simulink model "BMS_V4"  (R2017b)
settings: Solver=FixedStepDiscrete  StartTime=0.0  StopTime=inf  FixedStep=BASETIME  RelTol=1e-3  EnableMultiTasking=on
values from neighbouring files (symbols this model uses):
  AKT_BALANCE = uint16(8)    [BMS_V4_config.m]
  BALANCE = uint16(4)    [BMS_V4_config.m]
  BALANCE_RESISTOR = int32(5)    [BMS_V4_config.m]
  BALANCE_VEC = uint16(8)    [BMS_V4_config.m]
  CELL_SOC = uint16(7)    [BMS_V4_config.m]
  CELL_STATE = uint16(3)    [BMS_V4_config.m]
  CELL_TEMPERATURE = uint16(6)    [BMS_V4_config.m]
  CELL_VOLTAGE = uint16(5)    [BMS_V4_config.m]
  CELLACTBITFIELD = hex2dec('300')    [BMS_V4_config.m]
  CELLDEACTBITFIELD = hex2dec('100')    [BMS_V4_config.m]
  CELLT_BURST = uint16(6)    [BMS_V4_config.m]
  CELLV_BURST = uint16(5)    [BMS_V4_config.m]
  CLK_CYC_timer_1 = 586    [BMS_V4_config.m]
  CLK_CYC_timer_2 = 5860    [BMS_V4_config.m]
  CLK_CYC_timer_3 = 280    [BMS_V4_config.m]
  CLK_CYC_timer_4 = 586*100    (= 58600)    [BMS_V4_config.m]
  CLK_CYC_timer_5 = 5800*2    (= 11600)    [BMS_V4_config.m]
  CLK_CYC_timer_6 = 320    [BMS_V4_config.m]
  CN_CELLS = int32(40*3600)    [BMS_V4_config.m]
  CONTACTOR = uint16(1)    [BMS_V4_config.m]
  CONTACTOR_LOCKED = uint16(0)    [BMS_V4_config.m]
  CONTACTOR_UNLOCKED = uint16(1)    [BMS_V4_config.m]
  DEBUG_SEND_STATES = uint16(hex2dec('01'))    [BMS_V4_config.m]
  DELTA_SOC_BALANCE = int32(5*1e6)    [BMS_V4_config.m]
  DELTA_SOC_BALANCE_OFF = int32(1*1e5)    [BMS_V4_config.m]
  DETERMINE_MODEL_PARAMETER_ACT = uint16(100)    [BMS_V4_config.m]
  DETERMINE_MODEL_PARAMETER_SCC = uint16(101)    [BMS_V4_config.m]
  ERROR = uint16(1)    [BMS_V4_config.m]
  EXTERN_SIGNALS = uint16(1)    [BMS_V4_config.m]
  FREQUENCY_STEPS = uint16([25 50 75 100 150 250 500 750                                      1000 1500 2500 5000 7500                                      10010 10015 10025 10050 10075                                      10100 10150 10250 10500 10750                                      11000 11500])    [BMS_V4_config.m]
  GET_IMAG_PART_MFC = uint16(9)    [BMS_V4_config.m]
  GET_IMAG_PART_MSF = uint16(4)    [BMS_V4_config.m]
  GET_REAL_PART_MFC = uint16(8)    [BMS_V4_config.m]
  GET_REAL_PART_MSF = uint16(3)    [BMS_V4_config.m]
  IMU = uint16(7)    [BMS_V4_config.m]
  IMU_AMP_OFF = uint16(5)    [BMS_V4_config.m]
  IMU_DATA_READ_LOCUS_ACT = uint16(6)    [BMS_V4_config.m]
  IMU_DATA_READ_LOCUS_SCC = uint16(7)    [BMS_V4_config.m]
  IMU_DEBUG = uint16(9)    [BMS_V4_config.m]
  IMU_GET_DATA_MFC = uint16(8)    [BMS_V4_config.m]
  IMU_GET_DATA_MSF = uint16(3)    [BMS_V4_config.m]
  IMU_OFFSET_POLLING = uint16(11)    [BMS_V4_config.m]
  IMU_POLLING = uint16(2)    [BMS_V4_config.m]
  IMU_POWER = uint16(10)    [BMS_V4_config.m]
  IMU_SEND_IMAG = uint16(11)    [BMS_V4_config.m]
  IMU_SEND_REAL = uint16(10)    [BMS_V4_config.m]
  INDEX_IMAGPART = uint16(2)    [BMS_V4_config.m]
  INDEX_REALPART = uint16(1)    [BMS_V4_config.m]
  INFO = uint16(2)    [BMS_V4_config.m]
  INIT_OFFSET_AMPLITUDE = uint16(2)    [BMS_V4_config.m]
  LINE_CURRENT = uint16(3)    [BMS_V4_config.m]
  LINE_CURRENT_CANA = uint16(4)    [BMS_V4_config.m]
  LINE_CURRENT_SWITCH_THRESHOLD = int32(2*1e6)    [BMS_V4_config.m]
  NUM_OF_CELLS = uint16(16)    [BMS_V4_config.m]
  NUM_OF_FREQUENCIES_PSO = uint16(14)    [BMS_V4_config.m]
  NUM_OF_LINES = uint16(1)    [BMS_V4_config.m]
  NUM_OF_PARAMETER = single(5)    [BMS_V4_config.m]
  NUM_OF_SOC_POINTS = uint16(110)    [BMS_V4_config.m]
  P_L_BOUND = single([0.05;0.01;0.1;0.01;0.1])    [BMS_V4_config.m]
  P_U_BOUND = single([0.50;0.20;0.9;0.06;60])    [BMS_V4_config.m]
  PARA_ACT_SEND = uint16(101)    [BMS_V4_config.m]
  PARA_DATA_STORE_ACT = uint16(8)    [BMS_V4_config.m]
  PARA_DATA_STORE_SCC = uint16(9)    [BMS_V4_config.m]
  PARA_SCC_SEND = uint16(102)    [BMS_V4_config.m]
  PARTICLE_INIT = single(create_startparticle(P_L_BOUND,P_U_BOUND,NUM_OF_PARTICLE))    [BMS_V4_config.m]
  POLACT = hex2dec('00000BFF')    [BMS_V4_config.m]
  POLDEACT = hex2dec('000008FF')    [BMS_V4_config.m]
  PSO_PARA_DEBUG = uint16(13)    [BMS_V4_config.m]
  REQUEST_SOC_REF = uint16(1000)    [BMS_V4_config.m]
  SCALE_FACTOR_CH1 = single(0.66666666)    [BMS_V4_config.m]
  SCALE_FACTOR_CH2 = single(0.66666666)    [BMS_V4_config.m]
  SEND_CELL_SOC_ABS = uint16(199)    [BMS_V4_config.m]
  SHUT_DOWN_BALANCE_OFF = uint16(3)    [BMS_V4_config.m]
  SHUT_DOWN_BALANCE_ON = uint16(2)    [BMS_V4_config.m]
  START_IMU_MSL = uint16(3)    [BMS_V4_config.m]
  START_IMU_SCC = uint16(1)    [BMS_V4_config.m]
  SWITCH_IMU_OFF = uint16(2)    [BMS_V4_config.m]
  SWITCH_IMU_ON = uint16(1)    [BMS_V4_config.m]
  SWITCH_IMU_ON_OFF = uint16(4)    [BMS_V4_config.m]
  SYSTEM_DEBUG = uint16(12)    [BMS_V4_config.m]
  TIMEOUT_CANA = uint32(5000)    [BMS_V4_config.m]
  TIMEOUT_GATEWAY = uint32(500)    [BMS_V4_config.m]
  TS_SOC = single(0.010)    [BMS_V4_config.m]
  WARNING = uint16(2)    [BMS_V4_config.m]
libraries: c280xlib x44, c2833xlib x5, simulink x2, c2000lib x1, idelinklib_common x1
(part 1 of 8)
settings Model: Creator=Rathmann  LastModifiedBy=Franke
settings DataIOCC: LimitDataPoints=on  SaveFormat=Array
settings OptimizationCC: DefaultUnderspecifiedDataType=single  LifeSpan=1  MaxStackSize=64
settings DebuggingCC: SolverPrmCheckMsg=warning  MultiTaskDSMMsg=warning  AllowSymbolicDim=off  SFUnexpectedBacktrackingDiag=warning  SFNoUnconditionalDefaultTransitionDiag=warning  SFExecutionAtInitializationDiag=none
settings HardwareCC: ProdBitPerChar=16  ProdBitPerInt=16  ProdBitPerPointer=16  ProdBitPerSizeT=32  ProdBitPerPtrDiffT=32  ProdLargestAtomicInteger=Integer  ProdLargestAtomicFloat=None  ProdWordSize=16  ProdHWDeviceType=Texas Instruments->C2000
settings ModelReferenceCC: PropagateSignalLabelsOutOfModel=off
settings SFSimCC: MATLABDynamicMemAlloc=off
settings RTWCC: SystemTargetFile=ert.tlc  HardwareBoard=TI Delfino F2833x (boot from flash)  TLCOptions=-aInlineSetEventsForThisBaseRateFcn=TLC_FALSE -aSuppressMultiTaskScheduler=TLC_FALSE -aRateBasedStepFcn=1  TemplateMakefile=ert_default_tmf  RTWVerbose=off  Toolchain=Texas Instruments Code Composer Studio (C2000)  BuildConfiguration=Faster Runs
settings CodeAppCC: IgnoreCustomStorageClasses=off  StateflowObjectComments=on
settings ERTTargetCC: CodeReplacementLibrary=TI C28x with C99 extensions  MultiwordLength=2048  CombineOutputUpdateFcns=off  ConvertIfToSwitch=off  SuppressUnreachableDefaultCases=off  MemSecPackage=mpt
settings ConfigComp: CovMetricSettings=dw  CovHtmlReporting=on  CovSaveCumulativeToWorkspaceVar=on  CovSaveSingleToWorkspaceVar=on  CovExternalEMLEnable=off  CovSFcnEnable=off

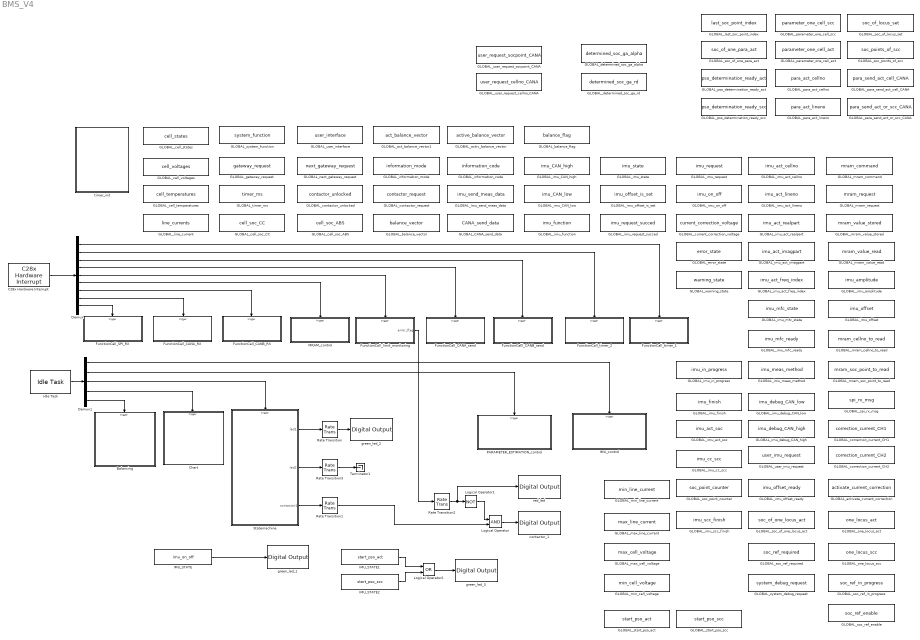
== system BMS_V4 ==
  Balancing : Stateflow chart  TreatAsAtomicUnit=on
  C28x Hardware Interrupt : c2000lib/Scheduling/C28x Hardware Interrupt  irqnumbers=[3 3 3 3 3 3 9 9 6]  pienumbers=[1 2 3 4 5 6 7 6 1]  irqpriorities=[36 37 38 39 30 41 35 34 33]  irqpreempts=[0 0 0 0 0 0 0 0 0]  showinput=off  dspchiptype=C280X
      settings: SourceProductName=Embedded Coder Support Package for Texas Instruments C2000 Processors  SourceProductBaseCode=TIC2000
  Chart : Stateflow chart  TreatAsAtomicUnit=on
  Demux : Demux  Outputs=9
  Demux1 : Demux  Outputs=5
  FunctionCall_CANA_RX : Subsystem  TreatAsAtomicUnit=on
      settings: RTWSystemCode=Nonreusable function  RTWFcnNameOpts=Use subsystem name  RTWFileNameOpts=Use subsystem name
  FunctionCall_CANA_send : Subsystem  TreatAsAtomicUnit=on
      settings: RTWSystemCode=Nonreusable function  RTWFcnNameOpts=Use subsystem name  RTWFileNameOpts=Use subsystem name
  FunctionCall_CANB_RX : Subsystem  TreatAsAtomicUnit=on
      settings: RTWSystemCode=Nonreusable function  RTWFcnNameOpts=Use subsystem name  RTWFileNameOpts=Use subsystem name  FunctionInterfaceSpec=Allow arguments
  FunctionCall_SPI_RX : Subsystem  TreatAsAtomicUnit=on
      settings: RTWSystemCode=Nonreusable function  RTWFcnNameOpts=Use subsystem name  RTWFileNameOpts=Use subsystem name
  FunctionCall_limit_monitoring : Stateflow chart  TreatAsAtomicUnit=on
      settings: RTWSystemCode=Nonreusable function  RTWFcnNameOpts=Use subsystem name  RTWFileNameOpts=Use subsystem name
  FunctionCall_timer_1 : Subsystem  TreatAsAtomicUnit=on
      settings: RTWSystemCode=Nonreusable function  RTWFcnNameOpts=Use subsystem name  RTWFileNameOpts=Use subsystem name
  FunctionCall_timer_2 : Subsystem  TreatAsAtomicUnit=on
      settings: RTWSystemCode=Nonreusable function  RTWFcnNameOpts=Use subsystem name  RTWFileNameOpts=Use subsystem name  FunctionInterfaceSpec=Allow arguments
  FunctionCalll_CANB_send : Subsystem  TreatAsAtomicUnit=on
      settings: RTWSystemCode=Nonreusable function  RTWFcnNameOpts=Use subsystem name  RTWFileNameOpts=Use subsystem name
  GLOBAL_CANA_send_data : DataStoreMemory  DataStoreName=CANA_send_data  ReadBeforeWriteMsg=warning  WriteAfterWriteMsg=warning  WriteAfterReadMsg=warning  InitialValue=CANA_SEND_DATA_INIT  ShowAdditionalParam=off  OutDataTypeStr=boolean
  GLOBAL_act_balance_vector1 : DataStoreMemory  DataStoreName=act_balance_vector  ReadBeforeWriteMsg=warning  WriteAfterWriteMsg=warning  WriteAfterReadMsg=warning  InitialValue=BALANCE_VECTOR_INIT  ShowAdditionalParam=off  OutDataTypeStr=boolean
  GLOBAL_activ_balance_vector : DataStoreMemory  DataStoreName=active_balance_vector  ReadBeforeWriteMsg=warning  WriteAfterWriteMsg=warning  WriteAfterReadMsg=warning  InitialValue=ACTIVE_BALANCE_VECTOR_INIT  ShowAdditionalParam=off  OutDataTypeStr=uint32
  GLOBAL_activate_current_correction : DataStoreMemory  DataStoreName=activate_current_correction  ReadBeforeWriteMsg=warning  WriteAfterWriteMsg=warning  WriteAfterReadMsg=warning  ShowAdditionalParam=off  OutDataTypeStr=boolean
  GLOBAL_balance_flag : DataStoreMemory  DataStoreName=balance_flag  ReadBeforeWriteMsg=warning  WriteAfterWriteMsg=warning  WriteAfterReadMsg=warning  InitialValue=BALANCE_FLAG_INIT  ShowAdditionalParam=off  OutDataTypeStr=boolean
  GLOBAL_balance_vector : DataStoreMemory  DataStoreName=balance_vector  ReadBeforeWriteMsg=warning  WriteAfterWriteMsg=warning  WriteAfterReadMsg=warning  InitialValue=BALANCE_VECTOR_INIT  ShowAdditionalParam=off  OutDataTypeStr=boolean
  GLOBAL_cell_soc_ABS : DataStoreMemory  DataStoreName=cell_soc_ABS  ReadBeforeWriteMsg=warning  WriteAfterWriteMsg=warning  WriteAfterReadMsg=warning  InitialValue=CELL_SOC_ABS_INIT  ShowAdditionalParam=off  OutDataTypeStr=int32
  GLOBAL_cell_soc_CC : DataStoreMemory  DataStoreName=cell_soc_CC  ReadBeforeWriteMsg=warning  WriteAfterWriteMsg=warning  WriteAfterReadMsg=warning  InitialValue=CELL_SOC_CC_INIT  ShowAdditionalParam=off  OutDataTypeStr=int32
  GLOBAL_cell_states : DataStoreMemory  DataStoreName=cell_states  ReadBeforeWriteMsg=warning  WriteAfterWriteMsg=warning  WriteAfterReadMsg=warning  InitialValue=CELL_STATES_INIT  ShowAdditionalParam=off  OutDataTypeStr=uint32  DataLoggingName=va
      settings: DataLoggingNameMode=Custom
  GLOBAL_cell_temperatures : DataStoreMemory  DataStoreName=cell_temperatures  ReadBeforeWriteMsg=warning  WriteAfterWriteMsg=warning  WriteAfterReadMsg=warning  InitialValue=CELL_TEMPERATURES_INIT  VectorParams1D=off  ShowAdditionalParam=off  OutDataTypeStr=int16
  GLOBAL_cell_voltages : DataStoreMemory  DataStoreName=cell_voltages  ReadBeforeWriteMsg=warning  WriteAfterWriteMsg=warning  WriteAfterReadMsg=warning  InitialValue=CELL_VOLTAGES_INIT  ShowAdditionalParam=off  OutDataTypeStr=uint16  DataLoggingName=va
      settings: DataLoggingNameMode=Custom
  GLOBAL_contactor_request : DataStoreMemory  DataStoreName=contactor_request  ReadBeforeWriteMsg=warning  WriteAfterWriteMsg=warning  WriteAfterReadMsg=warning  ShowAdditionalParam=off  OutDataTypeStr=boolean
  GLOBAL_contactor_unlocked : DataStoreMemory  DataStoreName=contactor_unlocked  ReadBeforeWriteMsg=warning  WriteAfterWriteMsg=warning  WriteAfterReadMsg=warning  ShowAdditionalParam=off  OutDataTypeStr=boolean
  GLOBAL_correction_current_CH1 : DataStoreMemory  DataStoreName=correction_current_CH1  ReadBeforeWriteMsg=warning  WriteAfterWriteMsg=warning  WriteAfterReadMsg=warning  InitialValue=CURRENT_CORRECTION_INIT  ShowAdditionalParam=off  OutDataTypeStr=single
  GLOBAL_correction_current_CH2 : DataStoreMemory  DataStoreName=correction_current_CH2  ReadBeforeWriteMsg=warning  WriteAfterWriteMsg=warning  WriteAfterReadMsg=warning  InitialValue=CURRENT_CORRECTION_INIT  ShowAdditionalParam=off  OutDataTypeStr=single
  GLOBAL_current_correction_voltage : DataStoreMemory  DataStoreName=current_correction_voltage  ReadBeforeWriteMsg=warning  WriteAfterWriteMsg=warning  WriteAfterReadMsg=warning  ShowAdditionalParam=off  OutDataTypeStr=uint16
  GLOBAL_determined_soc_ga_alpha : DataStoreMemory  DataStoreName=determined_soc_ga_alpha  ReadBeforeWriteMsg=warning  WriteAfterWriteMsg=warning  WriteAfterReadMsg=warning  InitialValue=DETERMINED_SOC_GA_INIT  ShowAdditionalParam=off  OutDataTypeStr=int32
  GLOBAL_determined_soc_ga_rd : DataStoreMemory  DataStoreName=determined_soc_ga_rd  ReadBeforeWriteMsg=warning  WriteAfterWriteMsg=warning  WriteAfterReadMsg=warning  InitialValue=DETERMINED_SOC_GA_INIT  ShowAdditionalParam=off  OutDataTypeStr=int32
  GLOBAL_error_state : DataStoreMemory  DataStoreName=error_state  ReadBeforeWriteMsg=warning  WriteAfterWriteMsg=warning  WriteAfterReadMsg=warning  InitialValue=[0 0]  ShowAdditionalParam=off  OutDataTypeStr=uint16
  GLOBAL_gateway_request : DataStoreMemory  DataStoreName=gateway_request  ReadBeforeWriteMsg=warning  WriteAfterWriteMsg=warning  WriteAfterReadMsg=warning  InitialValue=GATEWAY_REQUEST_INIT  ShowAdditionalParam=off  OutDataTypeStr=boolean
  GLOBAL_imu_CAN_high : DataStoreMemory  DataStoreName=imu_CAN_high  ReadBeforeWriteMsg=warning  WriteAfterWriteMsg=warning  WriteAfterReadMsg=warning  ShowAdditionalParam=off  OutDataTypeStr=uint32
  GLOBAL_imu_CAN_low : DataStoreMemory  DataStoreName=imu_CAN_low  ReadBeforeWriteMsg=warning  WriteAfterWriteMsg=warning  WriteAfterReadMsg=warning  ShowAdditionalParam=off  OutDataTypeStr=uint32
  GLOBAL_imu_act_cellno : DataStoreMemory  DataStoreName=imu_act_cellno  ReadBeforeWriteMsg=warning  WriteAfterWriteMsg=warning  WriteAfterReadMsg=warning  InitialValue=1  ShowAdditionalParam=off  OutDataTypeStr=uint16
  GLOBAL_imu_act_freq_index : DataStoreMemory  DataStoreName=imu_act_freq_index  ReadBeforeWriteMsg=warning  WriteAfterWriteMsg=warning  WriteAfterReadMsg=warning  InitialValue=1  ShowAdditionalParam=off  OutDataTypeStr=uint16
  GLOBAL_imu_act_imagpart : DataStoreMemory  DataStoreName=imu_act_imagpart  ReadBeforeWriteMsg=warning  WriteAfterWriteMsg=warning  WriteAfterReadMsg=warning  ShowAdditionalParam=off  OutDataTypeStr=single
  GLOBAL_imu_act_lineno : DataStoreMemory  DataStoreName=imu_act_lineno  ReadBeforeWriteMsg=warning  WriteAfterWriteMsg=warning  WriteAfterReadMsg=warning  InitialValue=1  ShowAdditionalParam=off  OutDataTypeStr=uint16
  GLOBAL_imu_act_realpart : DataStoreMemory  DataStoreName=imu_act_realpart  ReadBeforeWriteMsg=warning  WriteAfterWriteMsg=warning  WriteAfterReadMsg=warning  ShowAdditionalParam=off  OutDataTypeStr=single
  GLOBAL_imu_act_soc : DataStoreMemory  DataStoreName=imu_act_soc  ReadBeforeWriteMsg=warning  WriteAfterWriteMsg=warning  WriteAfterReadMsg=warning  ShowAdditionalParam=off  OutDataTypeStr=int32
  GLOBAL_imu_amplitude : DataStoreMemory  DataStoreName=imu_amplitude  ReadBeforeWriteMsg=warning  WriteAfterWriteMsg=warning  WriteAfterReadMsg=warning  InitialValue=IMU_AMPLITUDE_INIT  ShowAdditionalParam=off  OutDataTypeStr=uint16
  GLOBAL_imu_cc_scc : DataStoreMemory  DataStoreName=imu_cc_scc  ReadBeforeWriteMsg=warning  WriteAfterWriteMsg=warning  WriteAfterReadMsg=warning  InitialValue=IMU_CC_SCC_INIT  ShowAdditionalParam=off  OutDataTypeStr=int32
  GLOBAL_imu_debug_CAN_high : DataStoreMemory  DataStoreName=imu_debug_CAN_high  ReadBeforeWriteMsg=warning  WriteAfterWriteMsg=warning  WriteAfterReadMsg=warning  ShowAdditionalParam=off  OutDataTypeStr=uint32
  GLOBAL_imu_debug_CAN_low : DataStoreMemory  DataStoreName=imu_debug_CAN_low  ReadBeforeWriteMsg=warning  WriteAfterWriteMsg=warning  WriteAfterReadMsg=warning  ShowAdditionalParam=off  OutDataTypeStr=uint32
  GLOBAL_imu_finish : DataStoreMemory  DataStoreName=imu_finish  ReadBeforeWriteMsg=warning  WriteAfterWriteMsg=warning  WriteAfterReadMsg=warning  InitialValue=false  ShowAdditionalParam=off  OutDataTypeStr=boolean
  GLOBAL_imu_function : DataStoreMemory  DataStoreName=imu_function  ReadBeforeWriteMsg=warning  WriteAfterWriteMsg=warning  WriteAfterReadMsg=warning  InitialValue=IMU_FUNCTION_INIT  ShowAdditionalParam=off  OutDataTypeStr=uint16
  GLOBAL_imu_in_progress : DataStoreMemory  DataStoreName=imu_in_progress  ReadBeforeWriteMsg=warning  WriteAfterWriteMsg=warning  WriteAfterReadMsg=warning  ShowAdditionalParam=off  OutDataTypeStr=boolean
  GLOBAL_imu_meas_method : DataStoreMemory  DataStoreName=imu_meas_method  ReadBeforeWriteMsg=warning  WriteAfterWriteMsg=warning  WriteAfterReadMsg=warning  InitialValue=IMU_MEAS_METHOD_INIT  ShowAdditionalParam=off  OutDataTypeStr=uint16
  GLOBAL_imu_mfc_ready : DataStoreMemory  DataStoreName=imu_mfc_ready  ReadBeforeWriteMsg=warning  WriteAfterWriteMsg=warning  WriteAfterReadMsg=warning  ShowAdditionalParam=off  OutDataTypeStr=boolean
  GLOBAL_imu_mfc_state : DataStoreMemory  DataStoreName=imu_mfc_state  ReadBeforeWriteMsg=warning  WriteAfterWriteMsg=warning  WriteAfterReadMsg=warning  ShowAdditionalParam=off  OutDataTypeStr=uint16
  GLOBAL_imu_offset : DataStoreMemory  DataStoreName=imu_offset  ReadBeforeWriteMsg=warning  WriteAfterWriteMsg=warning  WriteAfterReadMsg=warning  InitialValue=IMU_OFFSET_INIT  ShowAdditionalParam=off  OutDataTypeStr=uint16
  GLOBAL_imu_offset_is_set : DataStoreMemory  DataStoreName=imu_offset_is_set  ReadBeforeWriteMsg=warning  WriteAfterWriteMsg=warning  WriteAfterReadMsg=warning  ShowAdditionalParam=off  OutDataTypeStr=boolean
  GLOBAL_imu_offset_ready : DataStoreMemory  DataStoreName=imu_offset_ready  ReadBeforeWriteMsg=warning  WriteAfterWriteMsg=warning  WriteAfterReadMsg=warning  ShowAdditionalParam=off  OutDataTypeStr=boolean
  GLOBAL_imu_on_off : DataStoreMemory  DataStoreName=imu_on_off  ReadBeforeWriteMsg=warning  WriteAfterWriteMsg=warning  WriteAfterReadMsg=warning  ShowAdditionalParam=off  OutDataTypeStr=boolean
  GLOBAL_imu_request : DataStoreMemory  DataStoreName=imu_request  ReadBeforeWriteMsg=warning  WriteAfterWriteMsg=warning  WriteAfterReadMsg=warning  ShowAdditionalParam=off  OutDataTypeStr=uint16
  GLOBAL_imu_request_succed : DataStoreMemory  DataStoreName=imu_request_succed  ReadBeforeWriteMsg=warning  WriteAfterWriteMsg=warning  WriteAfterReadMsg=warning  ShowAdditionalParam=off  OutDataTypeStr=boolean
  GLOBAL_imu_scc_finish : DataStoreMemory  DataStoreName=imu_scc_finish  ReadBeforeWriteMsg=warning  WriteAfterWriteMsg=warning  WriteAfterReadMsg=warning  InitialValue=false  ShowAdditionalParam=off  OutDataTypeStr=boolean
  GLOBAL_imu_send_meas_data : DataStoreMemory  DataStoreName=imu_send_meas_data  ReadBeforeWriteMsg=warning  WriteAfterWriteMsg=warning  WriteAfterReadMsg=warning  ShowAdditionalParam=off  OutDataTypeStr=boolean
  GLOBAL_imu_state : DataStoreMemory  DataStoreName=imu_state  ReadBeforeWriteMsg=warning  WriteAfterWriteMsg=warning  WriteAfterReadMsg=warning  ShowAdditionalParam=off  OutDataTypeStr=uint16
  GLOBAL_information_code : DataStoreMemory  DataStoreName=information_code  ReadBeforeWriteMsg=warning  WriteAfterWriteMsg=warning  WriteAfterReadMsg=warning  ShowAdditionalParam=off  OutDataTypeStr=uint16
  GLOBAL_information_mode : DataStoreMemory  DataStoreName=information_mode  ReadBeforeWriteMsg=warning  WriteAfterWriteMsg=warning  WriteAfterReadMsg=warning  InitialValue=EXTERN_SIGNALS  ShowAdditionalParam=off  OutDataTypeStr=uint16
  GLOBAL_last_soc_point_index : DataStoreMemory  DataStoreName=last_soc_point_index  ReadBeforeWriteMsg=warning  WriteAfterWriteMsg=warning  WriteAfterReadMsg=warning  InitialValue=LAST_SOC_POINT_INDEX_INIT  ShowAdditionalParam=off  OutDataTypeStr=uint16
  GLOBAL_line_current : DataStoreMemory  DataStoreName=line_currents  ReadBeforeWriteMsg=warning  WriteAfterWriteMsg=warning  WriteAfterReadMsg=warning  InitialValue=LINE_CURRENT_INIT  ShowAdditionalParam=off  OutDataTypeStr=int32
  GLOBAL_max_cell_voltage : DataStoreMemory  DataStoreName=max_cell_voltage  ReadBeforeWriteMsg=warning  WriteAfterWriteMsg=warning  WriteAfterReadMsg=warning  InitialValue=MAX_CELL_VOLTAGE_INIT  ShowAdditionalParam=off  OutDataTypeStr=uint16
  GLOBAL_max_line_current : DataStoreMemory  DataStoreName=max_line_current  ReadBeforeWriteMsg=warning  WriteAfterWriteMsg=warning  WriteAfterReadMsg=warning  ShowAdditionalParam=off  OutDataTypeStr=int32
  GLOBAL_min_cell_voltage : DataStoreMemory  DataStoreName=min_cell_voltage  ReadBeforeWriteMsg=warning  WriteAfterWriteMsg=warning  WriteAfterReadMsg=warning  InitialValue=MIN_CELL_VOLTAGE_INIT  ShowAdditionalParam=off  OutDataTypeStr=uint16
  GLOBAL_min_line_current : DataStoreMemory  DataStoreName=min_line_current  ReadBeforeWriteMsg=warning  WriteAfterWriteMsg=warning  WriteAfterReadMsg=warning  ShowAdditionalParam=off  OutDataTypeStr=int32
  GLOBAL_mram_cellno_to_read : DataStoreMemory  DataStoreName=mram_cellno_to_read  ReadBeforeWriteMsg=warning  WriteAfterWriteMsg=warning  WriteAfterReadMsg=warning  ShowAdditionalParam=off  OutDataTypeStr=uint16
  GLOBAL_mram_command : DataStoreMemory  DataStoreName=mram_command  ReadBeforeWriteMsg=warning  WriteAfterWriteMsg=warning  WriteAfterReadMsg=warning  InitialValue=MRAM_COMMAND_INIT  ShowAdditionalParam=off  OutDataTypeStr=boolean
  GLOBAL_mram_request : DataStoreMemory  DataStoreName=mram_request  ReadBeforeWriteMsg=warning  WriteAfterWriteMsg=warning  WriteAfterReadMsg=warning  InitialValue=uint16(0)  ShowAdditionalParam=off  OutDataTypeStr=uint16
  GLOBAL_mram_soc_point_to_read : DataStoreMemory  DataStoreName=mram_soc_point_to_read  ReadBeforeWriteMsg=warning  WriteAfterWriteMsg=warning  WriteAfterReadMsg=warning  ShowAdditionalParam=off  OutDataTypeStr=uint16
  GLOBAL_mram_value_read : DataStoreMemory  DataStoreName=mram_value_read  ReadBeforeWriteMsg=warning  WriteAfterWriteMsg=warning  WriteAfterReadMsg=warning  ShowAdditionalParam=off  OutDataTypeStr=boolean
  GLOBAL_mram_value_stored : DataStoreMemory  DataStoreName=mram_value_stored  ReadBeforeWriteMsg=warning  WriteAfterWriteMsg=warning  WriteAfterReadMsg=warning  ShowAdditionalParam=off  OutDataTypeStr=boolean
  GLOBAL_next_gateway_request : DataStoreMemory  DataStoreName=next_gateway_request  ReadBeforeWriteMsg=warning  WriteAfterWriteMsg=warning  WriteAfterReadMsg=warning  ShowAdditionalParam=off  OutDataTypeStr=boolean
  GLOBAL_one_locus_act : DataStoreMemory  DataStoreName=one_locus_act  ReadBeforeWriteMsg=warning  WriteAfterWriteMsg=warning  WriteAfterReadMsg=warning  InitialValue=ONE_LOCUS_INIT  ShowAdditionalParam=off  OutDataTypeStr=single
  GLOBAL_one_locus_scc : DataStoreMemory  DataStoreName=one_locus_scc  ReadBeforeWriteMsg=warning  WriteAfterWriteMsg=warning  WriteAfterReadMsg=warning  InitialValue=ONE_LOCUS_INIT  ShowAdditionalParam=off  OutDataTypeStr=single
  GLOBAL_para_act_cellno : DataStoreMemory  DataStoreName=para_act_cellno  ReadBeforeWriteMsg=warning  WriteAfterWriteMsg=warning  WriteAfterReadMsg=warning  InitialValue=1  ShowAdditionalParam=off  OutDataTypeStr=uint16
  GLOBAL_para_act_lineno : DataStoreMemory  DataStoreName=para_act_lineno  ReadBeforeWriteMsg=warning  WriteAfterWriteMsg=warning  WriteAfterReadMsg=warning  InitialValue=1  ShowAdditionalParam=off  OutDataTypeStr=uint16
  GLOBAL_para_send_act_cell_CANA : DataStoreMemory  DataStoreName=para_send_act_cell_CANA  ReadBeforeWriteMsg=warning  WriteAfterWriteMsg=warning  WriteAfterReadMsg=warning  InitialValue=1  ShowAdditionalParam=off  OutDataTypeStr=uint16
  GLOBAL_para_send_act_or_scc_CANA : DataStoreMemory  DataStoreName=para_send_act_or_scc_CANA  ReadBeforeWriteMsg=warning  WriteAfterWriteMsg=warning  WriteAfterReadMsg=warning  InitialValue=PARA_ACT_SEND  ShowAdditionalParam=off  OutDataTypeStr=uint16
  GLOBAL_parameter_one_cell_act : DataStoreMemory  DataStoreName=parameter_one_cell_act  ReadBeforeWriteMsg=warning  WriteAfterWriteMsg=warning  WriteAfterReadMsg=warning  InitialValue=PARAMETER_ONE_CELL_ACT_INIT  ShowAdditionalParam=off  OutDataTypeStr=single
  GLOBAL_parameter_one_cell_scc : DataStoreMemory  DataStoreName=parameter_one_cell_scc  ReadBeforeWriteMsg=warning  WriteAfterWriteMsg=warning  WriteAfterReadMsg=warning  InitialValue=PARAMETER_ONE_CELL_SCC_INIT  ShowAdditionalParam=off  OutDataTypeStr=single
  GLOBAL_pso_determination_ready_act : DataStoreMemory  DataStoreName=pso_determination_ready_act  ReadBeforeWriteMsg=warning  WriteAfterWriteMsg=warning  WriteAfterReadMsg=warning  ShowAdditionalParam=off  OutDataTypeStr=boolean
  GLOBAL_pso_determination_ready_scc : DataStoreMemory  DataStoreName=pso_determination_ready_scc  ReadBeforeWriteMsg=warning  WriteAfterWriteMsg=warning  WriteAfterReadMsg=warning  ShowAdditionalParam=off  OutDataTypeStr=boolean
  GLOBAL_soc_of_locus_set : DataStoreMemory  DataStoreName=soc_of_locus_set  ReadBeforeWriteMsg=warning  WriteAfterWriteMsg=warning  WriteAfterReadMsg=warning  InitialValue=SOC_OF_LOCUS_SET_INIT  ShowAdditionalParam=off  OutDataTypeStr=int32
  GLOBAL_soc_of_one_locus_act : DataStoreMemory  DataStoreName=soc_of_one_locus_act  ReadBeforeWriteMsg=warning  WriteAfterWriteMsg=warning  WriteAfterReadMsg=warning  InitialValue=SOC_OF_ONE_LOCUS_INIT  ShowAdditionalParam=off  OutDataTypeStr=int32
  GLOBAL_soc_of_one_para_act : DataStoreMemory  DataStoreName=soc_of_one_para_act  ReadBeforeWriteMsg=warning  WriteAfterWriteMsg=warning  WriteAfterReadMsg=warning  ShowAdditionalParam=off  OutDataTypeStr=int32
  GLOBAL_soc_point_counter : DataStoreMemory  DataStoreName=soc_point_counter  ReadBeforeWriteMsg=warning  WriteAfterWriteMsg=warning  WriteAfterReadMsg=warning  ShowAdditionalParam=off  OutDataTypeStr=uint16
  GLOBAL_soc_points_of_scc : DataStoreMemory  DataStoreName=soc_points_of_scc  ReadBeforeWriteMsg=warning  WriteAfterWriteMsg=warning  WriteAfterReadMsg=warning  InitialValue=SOC_POINTS_OF_SCC_INIT  ShowAdditionalParam=off  OutDataTypeStr=int32
  GLOBAL_soc_ref_enable : DataStoreMemory  DataStoreName=soc_ref_enable  ReadBeforeWriteMsg=warning  WriteAfterWriteMsg=warning  WriteAfterReadMsg=warning  ShowAdditionalParam=off  OutDataTypeStr=boolean
  GLOBAL_soc_ref_in_progress : DataStoreMemory  DataStoreName=soc_ref_in_progress  ReadBeforeWriteMsg=warning  WriteAfterWriteMsg=warning  WriteAfterReadMsg=warning  ShowAdditionalParam=off  OutDataTypeStr=boolean
  GLOBAL_soc_ref_required : DataStoreMemory  DataStoreName=soc_ref_required  ReadBeforeWriteMsg=warning  WriteAfterWriteMsg=warning  WriteAfterReadMsg=warning  ShowAdditionalParam=off  OutDataTypeStr=boolean
  GLOBAL_spi_rx_msg : DataStoreMemory  DataStoreName=spi_rx_msg  ReadBeforeWriteMsg=warning  WriteAfterWriteMsg=warning  WriteAfterReadMsg=warning  ShowAdditionalParam=off  OutDataTypeStr=uint32
  GLOBAL_start_pso_act : DataStoreMemory  DataStoreName=start_pso_act  ReadBeforeWriteMsg=warning  WriteAfterWriteMsg=warning  WriteAfterReadMsg=warning  InitialValue=false  ShowAdditionalParam=off  OutDataTypeStr=boolean
  GLOBAL_start_pso_scc : DataStoreMemory  DataStoreName=start_pso_scc  ReadBeforeWriteMsg=warning  WriteAfterWriteMsg=warning  WriteAfterReadMsg=warning  InitialValue=false  ShowAdditionalParam=off  OutDataTypeStr=boolean
  GLOBAL_system_debug_request : DataStoreMemory  DataStoreName=system_debug_request  ReadBeforeWriteMsg=warning  WriteAfterWriteMsg=warning  WriteAfterReadMsg=warning  ShowAdditionalParam=off  OutDataTypeStr=uint16
  GLOBAL_system_function : DataStoreMemory  DataStoreName=system_function  ReadBeforeWriteMsg=warning  WriteAfterWriteMsg=warning  WriteAfterReadMsg=warning  InitialValue=SYSTEM_FUNCTION_INIT  ShowAdditionalParam=off  OutDataTypeStr=boolean
  GLOBAL_timer_ms : DataStoreMemory  DataStoreName=timer_ms  ReadBeforeWriteMsg=warning  WriteAfterWriteMsg=warning  WriteAfterReadMsg=warning  ShowAdditionalParam=off  OutDataTypeStr=uint32
  GLOBAL_user_imu_request : DataStoreMemory  DataStoreName=user_imu_request  ReadBeforeWriteMsg=warning  WriteAfterWriteMsg=warning  WriteAfterReadMsg=warning  ShowAdditionalParam=off  OutDataTypeStr=uint16
  GLOBAL_user_interface : DataStoreMemory  DataStoreName=user_interface  ReadBeforeWriteMsg=warning  WriteAfterWriteMsg=warning  WriteAfterReadMsg=warning  InitialValue=USER_INTERFACE_INIT  ShowAdditionalParam=off  OutDataTypeStr=boolean
  GLOBAL_user_request_cellno_CANA : DataStoreMemory  DataStoreName=user_request_cellno_CANA  ReadBeforeWriteMsg=warning  WriteAfterWriteMsg=warning  WriteAfterReadMsg=warning  ShowAdditionalParam=off  OutDataTypeStr=uint16
  GLOBAL_user_request_socpoint_CANA : DataStoreMemory  DataStoreName=user_request_socpoint_CANA  ReadBeforeWriteMsg=warning  WriteAfterWriteMsg=warning  WriteAfterReadMsg=warning  ShowAdditionalParam=off  OutDataTypeStr=uint16
  GLOBAL_warning_state : DataStoreMemory  DataStoreName=warning_state  ReadBeforeWriteMsg=warning  WriteAfterWriteMsg=warning  WriteAfterReadMsg=warning  InitialValue=[0 0]  ShowAdditionalParam=off  OutDataTypeStr=uint16
  IMU_STATE : DataStoreRead  DataStoreName=imu_on_off
  IMU_STATE1 : DataStoreRead  DataStoreName=start_pso_act
  IMU_STATE2 : DataStoreRead  DataStoreName=start_pso_scc
  IMU_control : Stateflow chart  TreatAsAtomicUnit=on
      settings: RTWSystemCode=Nonreusable function  RTWFcnNameOpts=Use subsystem name  RTWFileNameOpts=Use subsystem name
  Idle Task : idelinklib_common/Idle Task  tasknumbers=[1 2 3 4 5]  taskpriorities=[100017 100018 100019 100020 100021]  taskpreempts=[0 1 0 1 1]  showinput=off  simPriority=0
  Logical Operator : Logic  AllPortsSameDT=off  OutDataTypeStr=boolean
  Logical Operator1 : Logic  Operator=NOT  AllPortsSameDT=off  OutDataTypeStr=boolean
  Logical Operator2 : Logic  Operator=OR  AllPortsSameDT=off  OutDataTypeStr=boolean
  MRAM_control : Stateflow chart  TreatAsAtomicUnit=on
      settings: RTWSystemCode=Nonreusable function  RTWFcnNameOpts=Use subsystem name  RTWFileNameOpts=Use subsystem name
  PARAMETER_ESTIMATION_control : Stateflow chart  TreatAsAtomicUnit=on
      settings: RTWSystemCode=Nonreusable function  RTWFcnNameOpts=Use subsystem name  RTWFileNameOpts=Use subsystem name
  Rate Transition{,1..3} (4 alike) : RateTransition  Deterministic=off  OutPortSampleTimeOpt=Inherit
  Statemachine : Stateflow chart  TreatAsAtomicUnit=on
      settings: RTWSystemCode=Nonreusable function  RTWFcnNameOpts=Use subsystem name  RTWFileNameOpts=Use subsystem name
  Terminator1 : Terminator
  contactor_1 : c2833xlib/Digital Output  GPIO_Number=GPIO0~GPIO7  GPIO_Bit0=off  GPIO_BIT0_Toggle=on  GPIO_Bit1=off  GPIO_BIT1_Toggle=off  GPIO_Bit2=off  GPIO_BIT2_Toggle=off  GPIO_Bit3=off  GPIO_BIT3_Toggle=off  GPIO_Bit4=off  GPIO_BIT4_Toggle=off  GPIO_Bit5=on  GPIO_BIT5_Toggle=off  GPIO_Bit6=off  GPIO_BIT6_Toggle=off  GPIO_Bit7=off  GPIO_BIT7_Toggle=off
      settings: SourceProductName=Embedded Coder Support Package for Texas Instruments C2000 Processors  SourceProductBaseCode=TIC2000
  green_led_1 : c2833xlib/Digital Output  GPIO_Number=GPIO0~GPIO7  GPIO_Bit0=on  GPIO_BIT0_Toggle=off  GPIO_Bit1=off  GPIO_BIT1_Toggle=off  GPIO_Bit2=off  GPIO_BIT2_Toggle=off  GPIO_Bit3=off  GPIO_BIT3_Toggle=off  GPIO_Bit4=off  GPIO_BIT4_Toggle=off  GPIO_Bit5=off  GPIO_BIT5_Toggle=off  GPIO_Bit6=off  GPIO_BIT6_Toggle=off  GPIO_Bit7=off  GPIO_BIT7_Toggle=off
      settings: SourceProductName=Embedded Coder Support Package for Texas Instruments C2000 Processors  SourceProductBaseCode=TIC2000
  green_led_2 : c2833xlib/Digital Output  GPIO_Number=GPIO0~GPIO7  GPIO_Bit0=off  GPIO_BIT0_Toggle=on  GPIO_Bit1=off  GPIO_BIT1_Toggle=off  GPIO_Bit2=on  GPIO_BIT2_Toggle=off  GPIO_Bit3=off  GPIO_BIT3_Toggle=off  GPIO_Bit4=off  GPIO_BIT4_Toggle=off  GPIO_Bit5=off  GPIO_BIT5_Toggle=off  GPIO_Bit6=off  GPIO_BIT6_Toggle=off  GPIO_Bit7=off  GPIO_BIT7_Toggle=off
      settings: SourceProductName=Embedded Coder Support Package for Texas Instruments C2000 Processors  SourceProductBaseCode=TIC2000
  green_led_3 : c2833xlib/Digital Output  GPIO_Number=GPIO0~GPIO7  GPIO_Bit0=off  GPIO_BIT0_Toggle=on  GPIO_Bit1=off  GPIO_BIT1_Toggle=off  GPIO_Bit2=off  GPIO_BIT2_Toggle=off  GPIO_Bit3=off  GPIO_BIT3_Toggle=off  GPIO_Bit4=on  GPIO_BIT4_Toggle=off  GPIO_Bit5=off  GPIO_BIT5_Toggle=off  GPIO_Bit6=off  GPIO_BIT6_Toggle=off  GPIO_Bit7=off  GPIO_BIT7_Toggle=off
      settings: SourceProductName=Embedded Coder Support Package for Texas Instruments C2000 Processors  SourceProductBaseCode=TIC2000
  red_led : c2833xlib/Digital Output  GPIO_Number=GPIO0~GPIO7  GPIO_Bit0=off  GPIO_BIT0_Toggle=on  GPIO_Bit1=off  GPIO_BIT1_Toggle=off  GPIO_Bit2=off  GPIO_BIT2_Toggle=off  GPIO_Bit3=off  GPIO_BIT3_Toggle=off  GPIO_Bit4=off  GPIO_BIT4_Toggle=off  GPIO_Bit5=off  GPIO_BIT5_Toggle=off  GPIO_Bit6=off  GPIO_BIT6_Toggle=off  GPIO_Bit7=on  GPIO_BIT7_Toggle=off
      settings: SourceProductName=Embedded Coder Support Package for Texas Instruments C2000 Processors  SourceProductBaseCode=TIC2000
  timer_init : Subsystem
  wires:
  C28x Hardware Interrupt/1 -> Demux/1
  Demux/2 -> FunctionCall_timer_2/Trigger
  Idle Task/1 -> Demux1/1
  Demux/7 -> FunctionCall_CANB_RX/Trigger
  Demux/4 -> FunctionCall_CANA_send/Trigger
  Demux/3 -> FunctionCalll_CANB_send/Trigger
  Demux/8 -> FunctionCall_CANA_RX/Trigger
  Demux/9 -> FunctionCall_SPI_RX/Trigger
  Statemachine/1(led1) -> Rate Transition/1
  Rate Transition/1 -> green_led_2/1
  Statemachine/3(contactor1) -> Rate Transition1/1
  IMU_STATE/1 -> green_led_1/1
  FunctionCall_limit_monitoring/1(error_flag) -> Rate Transition2/1
  Rate Transition1/1 -> Logical Operator/2
  Logical Operator/1 -> contactor_1/1
  Logical Operator1/1 -> Logical Operator/1
  Demux/1 -> FunctionCall_timer_1/Trigger
  Rate Transition2/1 -> red_led/1, Logical Operator1/1
  Demux/6 -> MRAM_control/Trigger
  Demux/5 -> FunctionCall_limit_monitoring/Trigger
  Demux1/1 -> IMU_control/Trigger
  Demux1/2 -> PARAMETER_ESTIMATION_control/Trigger
  Demux1/3 -> Statemachine/Trigger
  Statemachine/2(led2) -> Rate Transition3/1
  Rate Transition3/1 -> Terminator1/1
  IMU_STATE1/1 -> Logical Operator2/1
  IMU_STATE2/1 -> Logical Operator2/2
  Logical Operator2/1 -> green_led_3/1
  Demux1/4 -> Chart/Trigger
  Demux1/5 -> Balancing/Trigger

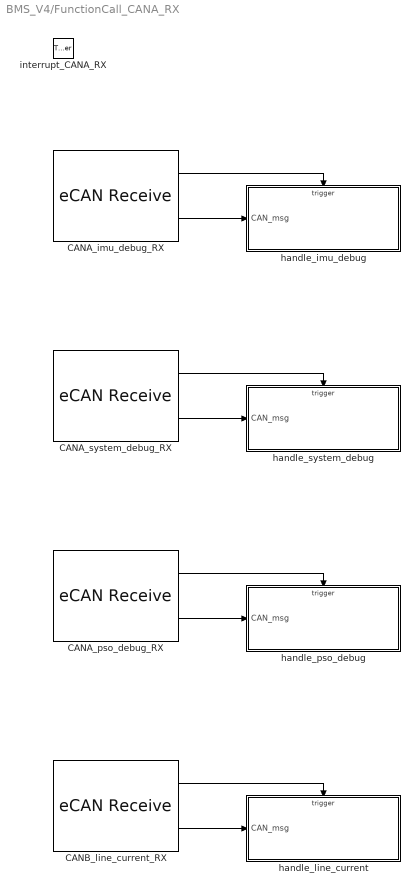
== system BMS_V4/FunctionCall_CANA_RX ==
  interrupt_CANA_RX : TriggerPort  TriggerType=function-call  VariantControl=Variant
  CANA_imu_debug_RX : c280xlib/eCAN Receive  chipFamily=C280x  useModule=eCAN_A  mailboxNo=23  messageID=ID_INIT_IMU_DEBUG  messageType=Standard (11-bit identifier)  sampleTime=-1  dataType=uint32  initValue=0  outputMessageLength=off  outputMessageTimeStamp=off  postInterrupt=on  interruptLine=1
      settings: SourceProductName=Embedded Coder Support Package for Texas Instruments C2000 Processors  SourceProductBaseCode=TIC2000
  CANA_pso_debug_RX : c280xlib/eCAN Receive  chipFamily=C280x  useModule=eCAN_A  mailboxNo=29  messageID=ID_INIT_PSO_DEBUG  messageType=Standard (11-bit identifier)  sampleTime=-1  dataType=uint32  initValue=0  outputMessageLength=off  outputMessageTimeStamp=off  postInterrupt=on  interruptLine=1
      settings: SourceProductName=Embedded Coder Support Package for Texas Instruments C2000 Processors  SourceProductBaseCode=TIC2000
  CANA_system_debug_RX : c280xlib/eCAN Receive  chipFamily=C280x  useModule=eCAN_A  mailboxNo=25  messageID=ID_INIT_SYSTEM_DEBUG  messageType=Standard (11-bit identifier)  sampleTime=-1  dataType=uint32  initValue=0  outputMessageLength=off  outputMessageTimeStamp=off  postInterrupt=on  interruptLine=1
      settings: SourceProductName=Embedded Coder Support Package for Texas Instruments C2000 Processors  SourceProductBaseCode=TIC2000
  CANB_line_current_RX : c280xlib/eCAN Receive  chipFamily=C280x  useModule=eCAN_A  mailboxNo=9  messageID=ID_LINE_CURRENT  messageType=Standard (11-bit identifier)  sampleTime=-1  dataType=uint32  initValue=0  outputMessageLength=off  outputMessageTimeStamp=off  postInterrupt=on  interruptLine=1
      settings: SourceProductName=Embedded Coder Support Package for Texas Instruments C2000 Processors  SourceProductBaseCode=TIC2000
  handle_imu_debug : Subsystem  TreatAsAtomicUnit=on
      settings: RTWSystemCode=Nonreusable function  RTWFcnNameOpts=Use subsystem name  RTWFileNameOpts=Use subsystem name
  handle_line_current : Subsystem  TreatAsAtomicUnit=on
      settings: RTWSystemCode=Nonreusable function  RTWFcnNameOpts=Use subsystem name  RTWFileNameOpts=Use subsystem name
  handle_pso_debug : Subsystem  TreatAsAtomicUnit=on
      settings: RTWSystemCode=Nonreusable function  RTWFcnNameOpts=Use subsystem name  RTWFileNameOpts=Use subsystem name
  handle_system_debug : Subsystem  TreatAsAtomicUnit=on
      settings: RTWSystemCode=Nonreusable function  RTWFcnNameOpts=Use subsystem name  RTWFileNameOpts=Use subsystem name
  wires:
  CANA_imu_debug_RX/1 -> handle_imu_debug/Trigger
  CANA_imu_debug_RX/2 -> handle_imu_debug/1(CAN_msg)
  CANA_system_debug_RX/1 -> handle_system_debug/Trigger
  CANA_system_debug_RX/2 -> handle_system_debug/1(CAN_msg)
  CANA_pso_debug_RX/1 -> handle_pso_debug/Trigger
  CANA_pso_debug_RX/2 -> handle_pso_debug/1(CAN_msg)
  CANB_line_current_RX/2 -> handle_line_current/1(CAN_msg)
  CANB_line_current_RX/1 -> handle_line_current/Trigger

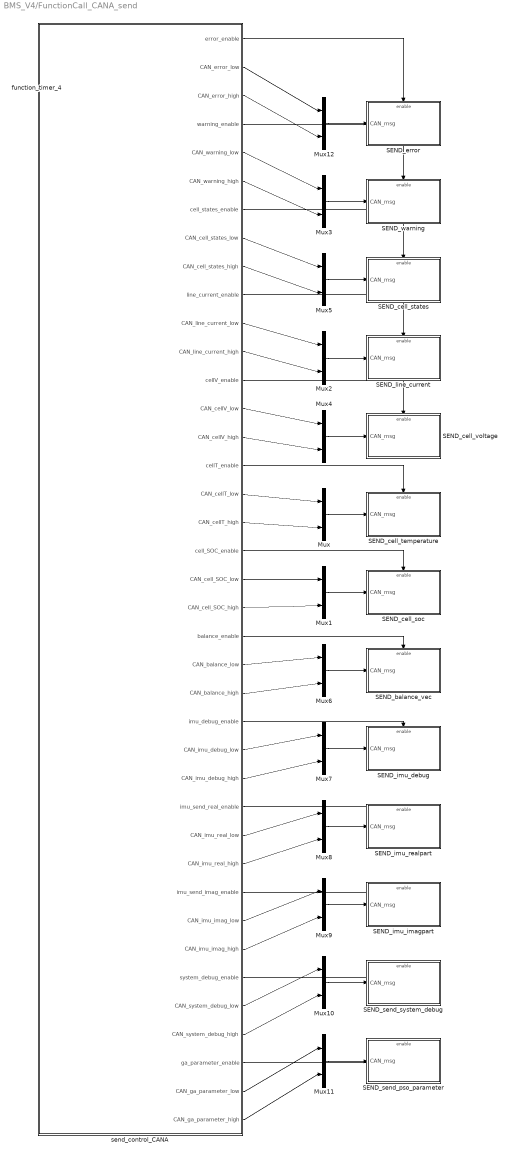
== system BMS_V4/FunctionCall_CANA_send ==
  function_timer_4 : TriggerPort  TriggerType=function-call  VariantControl=Variant
  Mux{,1..12} (13 alike) : Mux  Inputs=2
  SEND_balance_vec : Subsystem  TreatAsAtomicUnit=on
      settings: RTWSystemCode=Nonreusable function  RTWFcnNameOpts=Use subsystem name  RTWFileNameOpts=Use subsystem name
  SEND_cell_soc : Subsystem  TreatAsAtomicUnit=on
      settings: RTWSystemCode=Nonreusable function  RTWFcnNameOpts=Use subsystem name  RTWFileNameOpts=Use subsystem name
  SEND_cell_states : Subsystem  TreatAsAtomicUnit=on
      settings: RTWSystemCode=Nonreusable function  RTWFcnNameOpts=Use subsystem name  RTWFileNameOpts=Use subsystem name
  SEND_cell_temperature : Subsystem  TreatAsAtomicUnit=on
      settings: RTWSystemCode=Nonreusable function  RTWFcnNameOpts=Use subsystem name  RTWFileNameOpts=Use subsystem name
  SEND_cell_voltage : Subsystem  TreatAsAtomicUnit=on
      settings: RTWSystemCode=Nonreusable function  RTWFcnNameOpts=Use subsystem name  RTWFileNameOpts=Use subsystem name  FunctionInterfaceSpec=Allow arguments
  SEND_error : Subsystem  TreatAsAtomicUnit=on
      settings: RTWSystemCode=Nonreusable function  RTWFcnNameOpts=Use subsystem name  RTWFileNameOpts=Use subsystem name  FunctionInterfaceSpec=Allow arguments
  SEND_imu_debug : Subsystem  TreatAsAtomicUnit=on
      settings: RTWSystemCode=Nonreusable function  RTWFcnNameOpts=Use subsystem name  RTWFileNameOpts=Use subsystem name
  SEND_imu_imagpart : Subsystem  TreatAsAtomicUnit=on
      settings: RTWSystemCode=Nonreusable function  RTWFcnNameOpts=Use subsystem name  RTWFileNameOpts=Use subsystem name
  SEND_imu_realpart : Subsystem  TreatAsAtomicUnit=on
      settings: RTWSystemCode=Nonreusable function  RTWFcnNameOpts=Use subsystem name  RTWFileNameOpts=Use subsystem name
  SEND_line_current : Subsystem  TreatAsAtomicUnit=on
      settings: RTWSystemCode=Nonreusable function  RTWFcnNameOpts=Use subsystem name  RTWFileNameOpts=Use subsystem name
  SEND_send_pso_parameter : Subsystem  TreatAsAtomicUnit=on
      settings: RTWSystemCode=Nonreusable function  RTWFcnNameOpts=Use subsystem name  RTWFileNameOpts=Use subsystem name
  SEND_send_system_debug : Subsystem  TreatAsAtomicUnit=on
      settings: RTWSystemCode=Nonreusable function  RTWFcnNameOpts=Use subsystem name  RTWFileNameOpts=Use subsystem name
  SEND_warning : Subsystem  TreatAsAtomicUnit=on
      settings: RTWSystemCode=Nonreusable function  RTWFcnNameOpts=Use subsystem name  RTWFileNameOpts=Use subsystem name  FunctionInterfaceSpec=Allow arguments
  send_control_CANA : MATLAB Function  TreatAsAtomicUnit=on
      settings: RTWSystemCode=Nonreusable function  RTWFcnNameOpts=Use subsystem name  RTWFileNameOpts=Use subsystem name  FunctionInterfaceSpec=Allow arguments
  wires:
  Mux5/1 -> SEND_cell_states/1(CAN_msg)
  Mux4/1 -> SEND_cell_voltage/1(CAN_msg)
  Mux2/1 -> SEND_line_current/1(CAN_msg)
  Mux1/1 -> SEND_cell_soc/1(CAN_msg)
  Mux/1 -> SEND_cell_temperature/1(CAN_msg)
  Mux6/1 -> SEND_balance_vec/1(CAN_msg)
  send_control_CANA/22(balance_enable) -> SEND_balance_vec/Enable
  send_control_CANA/23(CAN_balance_low) -> Mux6/1
  send_control_CANA/24(CAN_balance_high) -> Mux6/2
  send_control_CANA/21(CAN_cell_SOC_high) -> Mux1/2
  send_control_CANA/20(CAN_cell_SOC_low) -> Mux1/1
  send_control_CANA/19(cell_SOC_enable) -> SEND_cell_soc/Enable
  send_control_CANA/16(cellT_enable) -> SEND_cell_temperature/Enable
  send_control_CANA/17(CAN_cellT_low) -> Mux/1
  send_control_CANA/18(CAN_cellT_high) -> Mux/2
  send_control_CANA/13(cellV_enable) -> SEND_cell_voltage/Enable
  send_control_CANA/14(CAN_cellV_low) -> Mux4/1
  send_control_CANA/15(CAN_cellV_high) -> Mux4/2
  send_control_CANA/10(line_current_enable) -> SEND_line_current/Enable
  send_control_CANA/11(CAN_line_current_low) -> Mux2/1
  send_control_CANA/12(CAN_line_current_high) -> Mux2/2
  send_control_CANA/8(CAN_cell_states_low) -> Mux5/1
  send_control_CANA/9(CAN_cell_states_high) -> Mux5/2
  send_control_CANA/7(cell_states_enable) -> SEND_cell_states/Enable
  send_control_CANA/5(CAN_warning_low) -> Mux3/1
  send_control_CANA/6(CAN_warning_high) -> Mux3/2
  Mux7/1 -> SEND_imu_debug/1(CAN_msg)
  send_control_CANA/25(imu_debug_enable) -> SEND_imu_debug/Enable
  send_control_CANA/26(CAN_imu_debug_low) -> Mux7/1
  send_control_CANA/27(CAN_imu_debug_high) -> Mux7/2
  Mux8/1 -> SEND_imu_realpart/1(CAN_msg)
  send_control_CANA/29(CAN_imu_real_low) -> Mux8/1
  send_control_CANA/30(CAN_imu_real_high) -> Mux8/2
  Mux9/1 -> SEND_imu_imagpart/1(CAN_msg)
  send_control_CANA/32(CAN_imu_imag_low) -> Mux9/1
  send_control_CANA/33(CAN_imu_imag_high) -> Mux9/2
  send_control_CANA/31(imu_send_imag_enable) -> SEND_imu_imagpart/Enable
  send_control_CANA/28(imu_send_real_enable) -> SEND_imu_realpart/Enable
  Mux10/1 -> SEND_send_system_debug/1(CAN_msg)
  send_control_CANA/34(system_debug_enable) -> SEND_send_system_debug/Enable
  send_control_CANA/35(CAN_system_debug_low) -> Mux10/1
  send_control_CANA/36(CAN_system_debug_high) -> Mux10/2
  Mux11/1 -> SEND_send_pso_parameter/1(CAN_msg)
  send_control_CANA/38(CAN_ga_parameter_low) -> Mux11/1
  send_control_CANA/39(CAN_ga_parameter_high) -> Mux11/2
  send_control_CANA/37(ga_parameter_enable) -> SEND_send_pso_parameter/Enable
  Mux3/1 -> SEND_warning/1(CAN_msg)
  send_control_CANA/4(warning_enable) -> SEND_warning/Enable
  send_control_CANA/1(error_enable) -> SEND_error/Enable
  send_control_CANA/2(CAN_error_low) -> Mux12/1
  send_control_CANA/3(CAN_error_high) -> Mux12/2
  Mux12/1 -> SEND_error/1(CAN_msg)

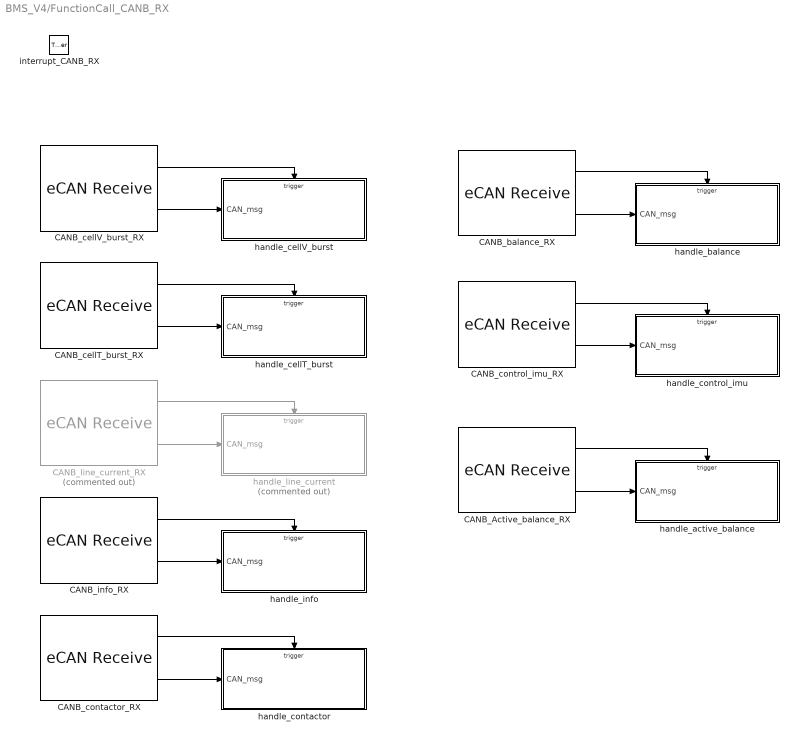
== system BMS_V4/FunctionCall_CANB_RX ==
  interrupt_CANB_RX : TriggerPort  TriggerType=function-call  VariantControl=Variant
  CANB_Active_balance_RX : c280xlib/eCAN Receive  chipFamily=C280x  useModule=eCAN_B  mailboxNo=15  messageID=ID_ACTIVE_BALANCE_ACK  messageType=Standard (11-bit identifier)  sampleTime=-1  dataType=uint32  initValue=0  outputMessageLength=off  outputMessageTimeStamp=off  postInterrupt=on  interruptLine=0
      settings: SourceProductName=Embedded Coder Support Package for Texas Instruments C2000 Processors  SourceProductBaseCode=TIC2000
  CANB_balance_RX : c280xlib/eCAN Receive  chipFamily=C280x  useModule=eCAN_B  mailboxNo=10  messageID=ID_BALANCE_ACK  messageType=Standard (11-bit identifier)  sampleTime=-1  dataType=uint32  initValue=0  outputMessageLength=off  outputMessageTimeStamp=off  postInterrupt=on  interruptLine=0
      settings: SourceProductName=Embedded Coder Support Package for Texas Instruments C2000 Processors  SourceProductBaseCode=TIC2000
  CANB_cellT_burst_RX : c280xlib/eCAN Receive  chipFamily=C280x  useModule=eCAN_B  mailboxNo=8  messageID=ID_CELLT_BURST  messageType=Standard (11-bit identifier)  sampleTime=-1  dataType=uint32  initValue=0  outputMessageLength=off  outputMessageTimeStamp=off  postInterrupt=on  interruptLine=0
      settings: SourceProductName=Embedded Coder Support Package for Texas Instruments C2000 Processors  SourceProductBaseCode=TIC2000
  CANB_cellV_burst_RX : c280xlib/eCAN Receive  chipFamily=C280x  useModule=eCAN_B  mailboxNo=7  messageID=ID_CELLV_BURST  messageType=Standard (11-bit identifier)  sampleTime=-1  dataType=uint32  initValue=0  outputMessageLength=off  outputMessageTimeStamp=off  postInterrupt=on  interruptLine=0
      settings: SourceProductName=Embedded Coder Support Package for Texas Instruments C2000 Processors  SourceProductBaseCode=TIC2000
  CANB_contactor_RX : c280xlib/eCAN Receive  chipFamily=C280x  useModule=eCAN_B  mailboxNo=12  messageID=ID_CONTACTOR  messageType=Standard (11-bit identifier)  sampleTime=-1  dataType=uint32  initValue=0  outputMessageLength=off  outputMessageTimeStamp=off  postInterrupt=on  interruptLine=0
      settings: SourceProductName=Embedded Coder Support Package for Texas Instruments C2000 Processors  SourceProductBaseCode=TIC2000
  CANB_control_imu_RX : c280xlib/eCAN Receive  chipFamily=C280x  useModule=eCAN_B  mailboxNo=14  messageID=ID_CONTROL_IMU  messageType=Standard (11-bit identifier)  sampleTime=-1  dataType=uint32  initValue=0  outputMessageLength=off  outputMessageTimeStamp=off  postInterrupt=on  interruptLine=0
      settings: SourceProductName=Embedded Coder Support Package for Texas Instruments C2000 Processors  SourceProductBaseCode=TIC2000
  CANB_info_RX : c280xlib/eCAN Receive  chipFamily=C280x  useModule=eCAN_B  mailboxNo=11  messageID=ID_INFO  messageType=Standard (11-bit identifier)  sampleTime=-1  dataType=uint32  initValue=0  outputMessageLength=off  outputMessageTimeStamp=off  postInterrupt=on  interruptLine=0
      settings: SourceProductName=Embedded Coder Support Package for Texas Instruments C2000 Processors  SourceProductBaseCode=TIC2000
  CANB_line_current_RX : c280xlib/eCAN Receive  Commented=on  chipFamily=C280x  useModule=eCAN_B  mailboxNo=9  messageID=ID_LINE_CURRENT  messageType=Standard (11-bit identifier)  sampleTime=-1  dataType=uint32  initValue=0  outputMessageLength=off  outputMessageTimeStamp=off  postInterrupt=on  interruptLine=0
      settings: SourceProductName=Embedded Coder Support Package for Texas Instruments C2000 Processors  SourceProductBaseCode=TIC2000
  handle_active_balance : Subsystem  TreatAsAtomicUnit=on
      settings: RTWSystemCode=Nonreusable function  RTWFcnNameOpts=Use subsystem name  RTWFileNameOpts=Use subsystem name
  handle_balance : Subsystem  TreatAsAtomicUnit=on
      settings: RTWSystemCode=Nonreusable function  RTWFcnNameOpts=Use subsystem name  RTWFileNameOpts=Use subsystem name
  handle_cellT_burst : Subsystem  TreatAsAtomicUnit=on
      settings: RTWSystemCode=Nonreusable function  RTWFcnNameOpts=Use subsystem name  RTWFileNameOpts=Use subsystem name
  handle_cellV_burst : Subsystem  TreatAsAtomicUnit=on
      settings: RTWSystemCode=Nonreusable function  RTWFcnNameOpts=Use subsystem name  RTWFileNameOpts=Use subsystem name  FunctionInterfaceSpec=Allow arguments
  handle_contactor : Subsystem  TreatAsAtomicUnit=on
      settings: RTWSystemCode=Nonreusable function  RTWFcnNameOpts=Use subsystem name  RTWFileNameOpts=Use subsystem name
  handle_control_imu : Subsystem  TreatAsAtomicUnit=on
      settings: RTWSystemCode=Nonreusable function  RTWFcnNameOpts=Use subsystem name  RTWFileNameOpts=Use subsystem name
  handle_info : Subsystem  TreatAsAtomicUnit=on
      settings: RTWSystemCode=Nonreusable function  RTWFcnNameOpts=Use subsystem name  RTWFileNameOpts=Use subsystem name
  handle_line_current : Subsystem  Commented=on  TreatAsAtomicUnit=on
      settings: RTWSystemCode=Nonreusable function  RTWFcnNameOpts=Use subsystem name  RTWFileNameOpts=Use subsystem name
  wires:
  CANB_cellV_burst_RX/2 -> handle_cellV_burst/1(CAN_msg)
  CANB_cellV_burst_RX/1 -> handle_cellV_burst/Trigger
  CANB_cellT_burst_RX/2 -> handle_cellT_burst/1(CAN_msg)
  CANB_cellT_burst_RX/1 -> handle_cellT_burst/Trigger
  CANB_line_current_RX/2 -> handle_line_current/1(CAN_msg)
  CANB_line_current_RX/1 -> handle_line_current/Trigger
  CANB_info_RX/2 -> handle_info/1(CAN_msg)
  CANB_info_RX/1 -> handle_info/Trigger
  CANB_contactor_RX/2 -> handle_contactor/1(CAN_msg)
  CANB_contactor_RX/1 -> handle_contactor/Trigger
  CANB_balance_RX/2 -> handle_balance/1(CAN_msg)
  CANB_balance_RX/1 -> handle_balance/Trigger
  CANB_control_imu_RX/2 -> handle_control_imu/1(CAN_msg)
  CANB_control_imu_RX/1 -> handle_control_imu/Trigger
  CANB_Active_balance_RX/2 -> handle_active_balance/1(CAN_msg)
  CANB_Active_balance_RX/1 -> handle_active_balance/Trigger

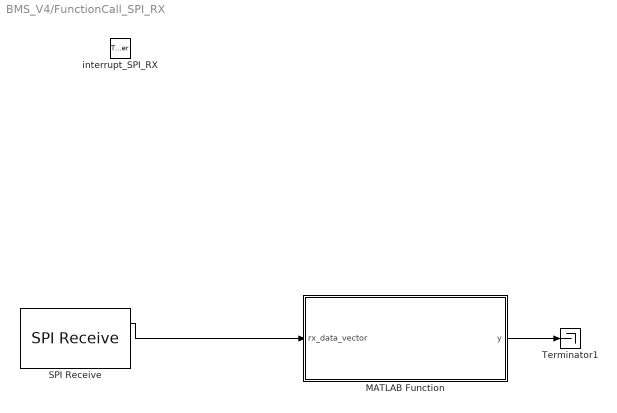
== system BMS_V4/FunctionCall_SPI_RX ==
  interrupt_SPI_RX : TriggerPort  TriggerType=function-call  VariantControl=Variant
  MATLAB Function : MATLAB Function  TreatAsAtomicUnit=on
  SPI Receive : c280xlib/SPI Receive  SPISelect=SPI_A  ClockPolarity=Falling_edge  ClockPhase=No_delay  SPIModule=uint32(0)  Mode=Master  BusSpeed=uint32(1000000)  FirstBitToTransfer=Most significant bit (MSB)  ClockMode=0  BlockFunction=Read  RegisterAddress=0  OutputDataType=uint16  OutputDataLength=8  BlockingMode=off  SampleTime=-1  DataBits=8  UseCustomSSPin=Provided by the SPI peripheral  ActiveLowSSPin=Active low  Pin=0
      settings: SourceProductName=Embedded Coder Support Package for Texas Instruments C2000 Processors  SourceProductBaseCode=TIC2000
  Terminator1 : Terminator
  wires:
  SPI Receive/1 -> MATLAB Function/1(rx_data_vector)
  MATLAB Function/1(y) -> Terminator1/1
